simulink model "FlightSimulation"  (R2025b)
settings: Solver=ode3  StartTime=0.0  StopTime=100  FixedStep=params.time.dt  RelTol=1e-3
values from neighbouring files (symbols this model uses):
  launch_ECEF_m = lla2ecef(launchLLA)    [RunSim.m]    (also in RunSimulink.m)
  launchAlt = 180    [RunSim.m]    (also in RunSimulink.m = 10)
  launchLLA = [launchLat, launchLon, launchAlt]    [RunSim.m]    (also in RunSimulink.m)
  q = q / norm(q)    [CorrectQuaternionKinematics.m]    (also in solveLQR.m = 0.5*rho*vel^2)
  q_TB_0 = dcm2quat(R_TB_0)    [RunSimulink.m]
  w_ib_x = 0.00    (= 0)    [RunSim.m]    (also in RunSimulink.m = 1e-10)
  w_ib_y = 0.00    (= 0)    [RunSim.m]    (also in RunSimulink.m = 1e-10)
  w_ib_z = 0.00    (= 0)    [RunSim.m]    (also in RunSimulink.m = 1e-10)
undefined symbols (not defined in the file or in its folder): Earth, F, kfConsts, kfErrInds, kfInds, launchGeoidHeight, Light, MIL, nav_covs, nav_state, params, WGS84, WMM2025
libraries: simulink x6, aerolibatmos2 x5, aerolibgravity2 x3, aerolib6dof2 x1, aerolibwind2 x1, simulink_extras x1, matrix_library x1, aerolibtransform2 x1, lib_utils x1
(part 2 of 2)

== system FlightSimulation/Flight Computer/UKF/Update Step/GPS Update ==
  SensorBus : Inport
  navBus : Inport  Port=2
  Enable : EnablePort
  Bus Selector : BusSelector  OutputSignals=MAX10S.P_T
  MATLAB Function : MATLAB Function  TreatAsAtomicUnit=on
  navOut : Outport
  wires:
  MATLAB Function/1(navOut) -> navOut/1
  navBus/1 -> MATLAB Function/1(navIn)
  SensorBus/1 -> Bus Selector/1
  Bus Selector/1 -> MATLAB Function/2(u_k)  "<P_T>"

== system FlightSimulation/Flight Computer/UKF/Update Step/Gravity Update ==
  navBus : Inport
  SensorBus : Inport  Port=2
  Enable : EnablePort
  Bus Selector : BusSelector  OutputSignals=ICM20948.sf_B_corr
  MATLAB Function : MATLAB Function  TreatAsAtomicUnit=on
  navOut : Outport
  wires:
  navBus/1 -> MATLAB Function/1(navIn)
  SensorBus/1 -> Bus Selector/1
  Bus Selector/1 -> MATLAB Function/2(accelMeas)  "<sf_B_corr>"
  MATLAB Function/1(navOut) -> navOut/1

== system FlightSimulation/Flight Computer/UKF/Update Step/Mag Update ==
  SensorBus : Inport
  navBus : Inport  Port=2
  Enable : EnablePort
  Bus Selector : BusSelector  OutputSignals=MMC5983.B_corr
  MATLAB Function : MATLAB Function  TreatAsAtomicUnit=on
  navOut : Outport
  wires:
  MATLAB Function/1(navOut) -> navOut/1
  navBus/1 -> MATLAB Function/1(navIn)
  SensorBus/1 -> Bus Selector/1
  Bus Selector/1 -> MATLAB Function/2(u_mag)  "<B_corr>"

== matlab function FlightSimulation/Flight Computer/InertialSensors/MATLAB Function1 ==
  data: u input; y output
function y = fcn(u)

y = u;

== matlab function FlightSimulation/Flight Computer/Sensor Bus/ICM20948/MATLAB Function ==
  data: a_b input; sf_true output; R_BT input
function sf_true = accel2sf_(a_b, R_BT)

sf_true = accel2sf(a_b, R_BT);

== matlab function FlightSimulation/Flight Computer/Sensor Bus/ICM20948/MATLAB Function 1 ==
  data: sf_true input; sf_corr output; rn input
function sf_corr = corruptSensorReading(sf_true, rn)

ICM20948_PARAMS = getICM20948Params();


sf_corr = applySensorModel(sf_true, ICM20948_PARAMS.accel, rn);

== matlab function FlightSimulation/Flight Computer/Sensor Bus/MATLAB Function1 ==
  data: B_true input; B_corr output; rn input
function B_corr = corruptSensorReading(B_true, rn)

MMC5983_PARAMS = getMMC5983Params();

B_corr = applySensorModel(B_true, MMC5983_PARAMS, rn);

== matlab function FlightSimulation/Flight Computer/UKF/Update Step/GPS Update/MATLAB Function ==
  data: navIn input Bus: kfParamsBus; navOut output Bus: kfParamsBus; kfInds parameter; kfErrInds parameter; kfConsts parameter; u_k input; time parameter
function navOut = gpsUpdate(navIn, kfInds, kfErrInds, kfConsts, u_k, time)

    % Force column
    u_k = u_k(:);
    navOut = navIn;

    %% === Setup ===
    x_pred = navOut.x;
    P_min  = navOut.P;

    % Measurement model: position only
    z = u_k(1:3);                  % GPS position measurement
    h = x_pred(kfInds.pos);        % Predicted position
    y = z - h;                     % Innovation

    %% === Measurement Jacobian wrt error state ===
    H = zeros(3, kfErrInds.maxStateIndex);
    H(:, kfErrInds.pos) = eye(3);  % Only sensitive to position errors

    %% === Kalman Update ===
    R = kfConsts.R_gps;  % Should be 3x3 covariance of GPS measurement
    S = H * P_min * H' + R;
    K = P_min * H' / S;

    dx = K * y;  % Error state correction

    %% === Apply Correction to Nominal State ===
    x_update = x_pred;

    % Apply additive position correction
    x_update(kfInds.pos) = x_update(kfInds.pos) + dx(kfErrInds.pos);

    % Optional: could add velocity or clock bias terms here if needed

    % Apply corrected state
    navOut.x = x_update;

    % Joseph form update (for stability)
    I = eye(size(P_min));
    navOut.P = I - K * H;
    navOut.P = navOut.P * P_min * navOut.P' + K * R * K';
    navOut.P = 0.5 * (navOut.P + navOut.P');  % Enforce symmetry

end

== matlab function FlightSimulation/Flight Computer/Perfect TRIAD, GPS/MATLAB Function ==
  data: newState output; PrevState input; new_pos input; new_q input
function newState = fcn(PrevState, new_pos, new_q)



newState = PrevState;
newState(8:10) = new_pos;
%disp(PrevState(1:4))

    newState(1:4) = new_q';

== matlab function FlightSimulation/Flight Computer/UKF/Update Step/Mag Update/MATLAB Function ==
  data: navIn input Bus: kfParamsBus; navOut output Bus: kfParamsBus; kfInds parameter; kfErrInds parameter; kfConsts parameter; u_mag input
function navOut = magHeadingUpdate(navIn, kfInds, kfErrInds, kfConsts, u_mag)
    navOut = navIn;

    %% === Setup ===
    x_pred = navOut.x;
    P_min  = navOut.P;

    q  = x_pred(kfInds.quat);         % [w x y z]
    bm = x_pred(kfInds.magBias);      % Magnetometer bias

    %% === Measured field in body frame (bias corrected, normalized)
    m_b = u_mag(:) - bm;
    m_b = m_b / norm(m_b + 1e-8);  % normalize with epsilon to avoid NaNs

    %% === Rotate to NED and project to horizontal plane
    R_BN = quat2rotm(q');             % Body-to-NED
    m_n = R_BN * m_b;
    m_n(3) = 0;

    if norm(m_n) < 1e-3
        return;  % Insufficient horizontal component to resolve heading
    end

    m_n = m_n / norm(m_n);
    yaw_meas = atan2(-m_n(2), m_n(1));  % Heading in NED frame (E/N)

    %% === Predicted yaw from current quaternion
    qw = q(1); qx = q(2); qy = q(3); qz = q(4);
    yaw_pred = atan2(2*(qw*qz + qx*qy), 1 - 2*(qy^2 + qz^2));

    %% === Innovation ===
    y = wrapToPi(yaw_meas - yaw_pred);

    %% === Jacobian: ∂yaw/∂(δθ)
    dq = 1e-5;
    H_theta = zeros(1, 3);
    for i = 1:3
        dtheta = zeros(3,1);
        dtheta(i) = dq;
        dq_pert = smallAngleQuaternion(dtheta);
        q_pert = quatmultiply(dq_pert', q')';
        R_pert = quat2rotm(q_pert');
        m_n_pert = R_pert * m_b;
        m_n_pert(3) = 0;
        if norm(m_n_pert) < 1e-3
            return;
        end
        m_n_pert = m_n_pert / norm(m_n_pert);
        yaw_pert = atan2(-m_n_pert(2), m_n_pert(1));
        H_theta(i) = (yaw_pert - yaw_pred) / dq;
    end

    %% === Jacobian: ∂yaw/∂(bm)
    H_bm = zeros(1, 3);
    for i = 1:3
        db = zeros(3,1);
        db(i) = dq;
        m_b_pert = (u_mag(:) - bm - db);  % Subtract db for ∂h/∂bm = -∂h/∂m_b
        m_b_pert = m_b_pert / norm(m_b_pert + 1e-8);
        m_n_pert = R_BN * m_b_pert;
        m_n_pert(3) = 0;
        if norm(m_n_pert) < 1e-3
            return;
        end
        m_n_pert = m_n_pert / norm(m_n_pert);
        yaw_pert = atan2(-m_n_pert(2), m_n_pert(1));
        H_bm(i) = (yaw_pert - yaw_pred) / dq;
    end

    %% === Assemble Kalman update ===
    H = zeros(1, kfErrInds.maxStateIndex);
    H(1, kfErrInds.theta) = H_theta;
    H(1, kfErrInds.magBias) = H_bm;

    R = deg2rad(3)^2;  % 3 deg stddev → variance

    S = H * P_min * H' + R;
    K = P_min * H' / S;
    dx = K * y;

    %% === Apply correction to nominal state ===
    delta_q = smallAngleQuaternion(dx(kfErrInds.theta));
    q_update = quatmultiply(delta_q', q')';
    q_update = q_update / norm(q_update);

    x_update = x_pred;
    x_update(kfInds.quat)     = q_update;
    x_update(kfInds.magBias)  = x_update(kfInds.magBias) + dx(kfErrInds.magBias);

    navOut.x = x_update;

    %% === Covariance Update (Joseph Form) ===
    I = eye(size(P_min));
    navOut.P = (I - K * H) * P_min * (I - K * H)' + K * R * K';
    navOut.P = 0.5 * (navOut.P + navOut.P');  % Force symmetry
end

== matlab function FlightSimulation/Flight Computer/Sensor Bus/MATLAB Function2 ==
  data: h input; P_true output; const parameter; P_corr output; geoid_height input; rn input
function [P_true, P_corr] = corruptBarometer(h, const, geoid_height, rn)

rng(42);

LPS22_PARAMS = getLPS22HHParams();

P_true = height2baro(h, geoid_height);

bias = LPS22_PARAMS.bias;
noise = LPS22_PARAMS.noise;
sf   = LPS22_PARAMS.sf;
k2   = LPS22_PARAMS.k2;
k3   = LPS22_PARAMS.k3;

P_corr = height2baro(h + bias + (noise * rn), geoid_height);

== matlab function FlightSimulation/Flight Computer/UKF/Update Step/Baro Update/MATLAB Function ==
  data: navIn input Bus: kfParamsBus; navOut output Bus: kfParamsBus; kfInds parameter; kfConsts parameter; u_baro input; const parameter
function navOut = magHeadingUpdate(navIn, kfInds, kfConsts, u_baro, const)
    navOut = navIn;

    if any(isnan(navOut.x_pred))
        navOut.x = navOut.x_pred;
        navOut.P = navOut.P_min;
        return;
    end

    %% === Setup ===
    x_pred = navOut.x;
    P_min  = navOut.P;

    % Convert Pressure to Altitude
    h_baro = (const.T0 / const.L) * (1 - (u_baro / const.P0)^(const.R * const.L / const.g_e));

    z_pred = x_pred(kfInds.pos(3));
    h_pred = -h_baro;

    % Innovation
    y = h_baro - h_pred;

    %% Measurement Jacobian
    H = zeros(1, length(x_pred));
    H(kfInds.pos(3)) = -1;

    % Measurement Noise
    R_baro = (0.3)^2; % [m]

    % Kalman Gain and Update
    S = H * P_min * H' + R_baro;
    K = P_min * H' / S;

    x_update = x_pred + K * y;
    navOut.x = x_update;

    P_update = (eye(length(x_pred)) - K * H) * P_min;
    navOut.P = 0.5 * (P_update + P_update');
    

end

== matlab function FlightSimulation/Flight Computer/Sensor Bus/ICM20948/MATLAB Function 2 ==
  data: gyro_true input; gyro_corr output; rn input
function gyro_corr = corruptSensorReading(gyro_true, rn)

ICM20948_PARAMS = getICM20948Params();


gyro_corr = applySensorModel(gyro_true, ICM20948_PARAMS.gyro, rn);

== matlab function FlightSimulation/Flight Computer/Perfect TRIAD, GPS/MATLAB Function1 ==
  data: u input; y output
function y = fcn(u)

y = u;

== matlab function FlightSimulation/Flight Computer/Perfect TRIAD, GPS/MATLAB Function2 ==
  data: a_b input; R_TB output; m_b input; a_i input; m_i input
function R_TB = fcn(a_b, m_b, a_i, m_i)
R_TB = computeInitialQuaternionTRIAD(a_b, m_b, a_i, m_i);

== matlab function FlightSimulation/Flight Computer/Perfect TRIAD, GPS/g->sf ==
  data: u input; y output
function y = fcn(u)

y = u;
y(3) = -1.0 * y(3);

== matlab function FlightSimulation/Flight Computer/UKF/Initialize Nav/Initialize State/MATLAB Function2 ==
  data: a_b input; q_0 output; m_b input
function q_0 = computeInitialQuaternion_(a_b, m_b)

    q_0 = NaN(4,1);

    if((norm(a_b) > 1))
        q_0(1:4) = computeInitialQuaternion(a_b, m_b);
    end

== matlab function FlightSimulation/Flight Computer/UKF/Initialize Nav/Initialize State/MATLAB Function3 ==
  data: initFlagLoop input; q_0 input; x_0 output; navInds parameter; navParams parameter; initFlag output
function [x_0, initFlag]= initializeState_(initFlagLoop, q_0, navInds, navParams)
%#codegen

    x_0 = navParams.x;

    if(initFlagLoop == 1)
        initFlag = 1;
        return;
    end

    if any(isnan(q_0))
        initFlag = 0;
    
    else 
        x_0(navInds.quat) = q_0;
        initFlag = 1;
    end

== stateflow chart FlightSimulation/Flight Computer/Nav State Machine/Chart ==
  state PreLaunch
  state Launch
    entry:
    state=1
    guid=0
  state Burnout
    entry:
    state=2
    guid=0
  state Guidance
    entry:
    state=3
    guid=1
  state Apogee
    entry:
    state=4
    guid=0
  (default) -> PreLaunch : {state=0}
  PreLaunch -> Launch : [A_b_x > 3]
  Launch -> Burnout : [A_b_x < 1]
  Burnout -> Guidance : [after(1, sec)]
  Guidance -> Apogee : [v_vert < 1]
  data: A_b_x input; alt input; v_vert input; guid output; state output

== matlab function FlightSimulation/Flight Computer/UKF/Update Step/Gravity Update/MATLAB Function ==
  data: navIn input Bus: kfParamsBus; navOut output Bus: kfParamsBus; kfInds parameter; kfErrInds parameter; kfConsts parameter; accelMeas input
function navOut = gravityUpdate(navIn, kfInds, kfErrInds, kfConsts, accelMeas)
    g = 9.80665;  % Gravity magnitude
    navOut = navIn;

    if any(isnan(navOut.x_pred))
        navOut.x = navOut.x_pred;
        navOut.P = navOut.P_min;
        return;
    end

    %% === Setup ===
    x_pred = navOut.x_pred;
    P_min  = navOut.P_min;

    q  = x_pred(kfInds.quat);        % Quaternion: body-to-NED
    ba = x_pred(kfInds.accelBias);   % Accel bias

    G_NED = [0; 0; g];               
    R_NB = quat2rotm(q');            % Rotation body-to-NED

    %% === Measurement Prediction ===
    accel_pred = R_NB' * G_NED + ba;
    accel_meas = accelMeas(:);
    
    % Optional: Skip update if dynamic
    if abs(norm(accel_meas) - g) > 1.0
        return;
    end

    y = accel_meas - accel_pred;

    %% === Jacobian ===
    H = zeros(3, kfErrInds.maxStateIndex);
    H(:, kfErrInds.theta)     = -R_NB * skew(G_NED);
    H(:, kfErrInds.accelBias) = eye(3);

    R = kfConsts.R_grav;

    %% === Kalman Update ===
    S = H * P_min * H' + R;
    K = P_min * H' / S;
    dx = K * y;

    %% === Apply Correction ===
    delta_theta = dx(kfErrInds.theta);
    angle = norm(delta_theta);
    if angle > deg2rad(10)
        delta_theta = delta_theta * (deg2rad(10) / angle);
    end

    delta_q = smallAngleQuaternion(delta_theta);
    q_update = quatmultiply(delta_q', q')';  % delta_q ⊗ q

    x_update = x_pred;
    x_update(kfInds.quat)       = q_update / norm(q_update);  
    x_update(kfInds.accelBias)  = x_update(kfInds.accelBias) + dx(kfErrInds.accelBias);

    %% === Covariance Update ===
    I = eye(size(P_min));
    P_update = (I - K * H) * P_min * (I - K * H)' + K * R * K'; 

    navOut.x = x_update;
    navOut.P = 0.5 * (P_update + P_update');  % Ensure symmetry
end

== matlab function FlightSimulation/Flight Computer/UKF/Update Step/MATLAB Function ==
  data: navOut output Bus: navBus; navIn input Bus: navBus
function navOut = passiveUpdate(navIn)

navOut = navIn;

navOut.x = navOut.x_min;
navOut.P = navOut.P_min;

navOut.P = (navOut.P + navOut.P') * 0.5;

== matlab function FlightSimulation/Flight Computer/Perfect TRIAD, GPS/Switch statement bruh why do i gotta make a matlab func for this ==
  data: a_b input; p_b output; a_i input; v_b input; v_i input; State input; p_i output
function [p_b, p_i] = fcn(a_b, a_i, v_b, v_i, State)
if State > 0 && State < 4
    p_b = v_b;
    p_i = v_i;
else
    p_b = a_b;
    p_i = a_i;
end

== matlab function FlightSimulation/Flight Computer/Perfect TRIAD, GPS/MATLAB Function3 ==
  data: u input; y output
function y = fcn(u)

y = [norm(u); 0; 0];

== matlab function FlightSimulation/Flight Computer/ESKF/GPS update ==
  settings: updateMethod=DISCRETE
  data: curr_state input; new_state output size=[20, 1]; curr_P input; State input; gps_pos_meas input; gps_vel_meas input; new_P output; time input
function [new_state, new_P] = fcn(curr_state, curr_P, State, gps_pos_meas, gps_vel_meas, time)
new_state = curr_state;
new_P = curr_P;


if (time > 0.1 && State ~= 1)
    GPS_PARAMS = getMAX10SParams();
    z = [gps_pos_meas; gps_vel_meas];
    h = [curr_state(8:10); curr_state(5:7)];
    H = [zeros(3, 6), eye(3, 3), zeros(3, 10);
        zeros(3, 3), eye(3, 3), zeros(3, 13)];
    R = diag([GPS_PARAMS.pos.noise; GPS_PARAMS.vel.noise]);
    
    [new_state, new_P] = residualErrInject(curr_state, curr_P, z, H, h, R);
end

end

== matlab function FlightSimulation/Flight Computer/ESKF/Accel+Mag update ==
  settings: updateMethod=DISCRETE
  data: curr_state input; new_state output; curr_P input; State input; accel_meas input; accel_inertial input; new_P output; mag_meas input; mag_inertial input; time input
function [new_state, new_P] = fcn(curr_state, curr_P, State, accel_meas, accel_inertial, mag_meas, mag_inertial, time)
new_state = curr_state;
new_P = curr_P;

MAG_PARAMS = getMMC5983Params();
ACCEL_PARAMS = getICM20948Params().accel;

q = curr_state(1:4)';

if (State == 0 && time > 0.1)

    rec_accel_body = quat2rotm(q)' * accel_inertial;
    rec_mag_body = quat2rotm(q)' * mag_inertial;
    
    
    z = [accel_meas; mag_meas];
    h = [rec_accel_body; rec_mag_body];
    H = [skewSymmetric(rec_accel_body), zeros(3, 9), eye(3, 3), zeros(3, 4);
        skewSymmetric(rec_mag_body), zeros(3, 12), eye(3, 3), zeros(3, 1)];
    R = diag([ACCEL_PARAMS.noise; MAG_PARAMS.noise]);
    
    [new_state, new_P] = residualErrInject(curr_state, curr_P, z, H, h, R);
else

end

== matlab function FlightSimulation/Flight Computer/ESKF/MATLAB Function2 ==
  data: a_b input; R_TB output; m_b input; a_i input; m_i input
function R_TB = fcn(a_b, m_b, a_i, m_i)
R_TB = computeInitialQuaternionTRIAD(a_b, m_b, a_i, m_i);

== matlab function FlightSimulation/Flight Computer/ESKF/MATLAB Function3 ==
  data: u input; y output
function y = fcn(u)

y = [norm(u); 0; 0];

== matlab function FlightSimulation/Flight Computer/UKF/Initialize Nav/Initialize State/MATLAB Function1 ==
  data: a_b input; eul_0 output; m_b input
function eul_0 = computeInitialOrientation_(a_b, m_b)

    % q_0 = NaN(4,1);
    eul_0 = NaN(3,1);

    if((norm(a_b) > 0.5))
        eul_0(1:3) = computeInitialOrientation(a_b, m_b);
    end

== matlab function FlightSimulation/Flight Computer/ESKF/Switch statement bruh why do i gotta make a matlab func for this ==
  data: a_b input; p_b output; a_i input; v_b input; v_i input; State input; p_i output
function [p_b, p_i] = fcn(a_b, a_i, v_b, v_i, State)
if State > 0 && State < 4
    p_b = v_b;
    p_i = v_i;
else
    p_b = a_b;
    p_i = a_i;
end

== matlab function FlightSimulation/Flight Computer/ESKF/g->sf ==
  data: u input; y output
function y = fcn(u)

y = u;
y(3) = -1.0 * y(3);

== matlab function FlightSimulation/Flight Computer/ESKF/Propagate non-linear dynamics aka fast gyro+accel prop ==
  data: gyro input; newState output; PrevState input; dt input; accel input; g_i input
function newState = fcn(gyro, PrevState, dt, accel, g_i)


prev_quat = quaternion(PrevState(1:4)');
prev_pos = PrevState(8:10);
prev_vel = PrevState(5:7);


newState = PrevState;

new_quat = propGyro(gyro, prev_quat, dt);
[new_pos, new_vel] = propAccel(accel, prev_vel, prev_pos, new_quat, g_i, dt);

newState(1:4) = new_quat;
newState(5:7) = new_vel;
newState(8:10) = new_pos;

== matlab function FlightSimulation/Flight Computer/ESKF/Predict Covs aka ekf predict ==
  settings: updateMethod=DISCRETE
  data: gyro input; curr_P output; accel input; prev_P input; curr_state input; dt input
function curr_P = fcn(gyro, accel, prev_P, curr_state, dt)

IMU_PARAMS = getICM20948Params();
MAG_PARAMS = getMMC5983Params();
BARO_PARAMS = getLPS22HHParams();


curr_quat = quaternion(curr_state(1:4)');

curr_P = predictCovariances(gyro, accel, prev_P, curr_quat, dt, IMU_PARAMS.gyro, IMU_PARAMS.accel, MAG_PARAMS, BARO_PARAMS);

== matlab function FlightSimulation/Flight Computer/ESKF/Baro update ==
  settings: updateMethod=DISCRETE
  data: curr_state input; new_state output; curr_P input size=[19, 19]; State input; baro_meas input; geoid_height input; launchAlt input; new_P output size=[19, 19]; time input; baro_height output
function [new_state, new_P, baro_height] = fcn(curr_state, curr_P, State, baro_meas, geoid_height, launchAlt, time)
new_state = curr_state;
new_P = curr_P;
baro_height = 0;

if (time > 0.1)
    BARO_PARAMS = getLPS22HHParams();
    
    baro_height = -1.0 * ((baro2height(baro_meas, geoid_height) - launchAlt) + curr_state(20));
    %disp("Baro height")
    %disp(time)
    %disp(baro_height)
    %disp("End")
    
    z = baro_height;
    h = [curr_state(10)];
    H = [zeros(1, 8), 1, zeros(1, 9), 1.0]; % TODO eventually add baro bias
    R = BARO_PARAMS.noise;
    [new_state, new_P] = residualErrInject(curr_state, curr_P, z, H, h, R);
end

end

== matlab function FlightSimulation/Flight Computer/ESKF/Unbias sensors ==
  data: w_ib_b_biased input; w_ib_b output; sf_b_biased input; B_biased input; LLA_biased input; V_T_biased input; P_biased input; prev_state input; sf_b output; B output; LLA output; V_T output; P output
function [w_ib_b, sf_b, B, LLA, V_T, P] = fcn(w_ib_b_biased, sf_b_biased, B_biased, LLA_biased, V_T_biased, P_biased, prev_state)

w_ib_b = w_ib_b_biased - prev_state(11:13);
sf_b = sf_b_biased - prev_state(14:16);
B = B_biased - prev_state(17:19);
LLA = LLA_biased;
V_T = V_T_biased;
%P = P_biased - prev_state(20);
P = P_biased;

== matlab function FlightSimulation/Flight Computer/UKF/Prediction Step/MATLAB Function ==
  data: navOut output Bus: navBus; navIn input Bus: navBus; sf_b input; w_ib_b input; time parameter; navInds parameter; navParams parameter
function navOut = UKFPredict(navIn, sf_b, w_ib_b, time, navInds, navParams)

dt = time.navDt;

% === Format Input ===
u = [w_ib_b(:); sf_b(:)];

navOut = navIn;

%% === GENERATE SIGMA POINTS ===
[X_sigma, P_sigma] = unscentedSigmaPoints(navIn.x, navIn.P, navParams.lambda);

X_sigma_pred = processModel(X_sigma, u, dt, navInds);

[x_min, P_min] = unscentedMeanCov(X_sigma_pred, navIn.W_m, navIn.W_c, navParams.Q);

navOut.x_min  = x_min;
navOut.P_min  = P_min;

% persistent ukf
% 
% if(isempty(ukf))
%     dynamicsFunc = @(x, dt, u) ukfDynamics(x, dt, u, navInds);
%     ukf = StavUKF(dynamicsFunc, navIn.Q);
% end
% 

% 
% % === Prepare State Struct ===
% stateStruct.mean = navIn.x;
% stateStruct.cov  = navIn.P;
% 
% % === UKF Prediction Step ===
% [prior, sigma] = ukf.predict(stateStruct, dt, u);
% 
% sigPts = sigma.sigmaPts;

% === Fill Output Bus ===
% navOut.x_min = prior.mean;
% navOut.P_min  = prior.cov;

== stateflow chart FlightSimulation/Flight Computer/State Machine/Chart ==
  state PreLaunch
  state Launch
    entry:
    state=1
    guid=0
  state Burnout
    entry:
    state=2
    guid=0
  state Guidance
    entry:
    state=3
    guid=1
  state Apogee
    entry:
    state=4
    guid=0
  (default) -> PreLaunch : {state=0}
  PreLaunch -> Launch : [A_b_x > 3]
  Launch -> Burnout : [A_b_x < 1]
  Burnout -> Guidance : [after(1, sec)]
  Guidance -> Apogee : [v_vert < 1]
  data: A_b_x input; alt input; v_vert input; guid output; state output; v_b input

== matlab function FlightSimulation/Flight Computer/UKF/Initialize Nav/Initialize State/MATLAB Function4 ==
  data: initFlagLoop input; eul_0 input; x_0 output; navInds parameter; navParams parameter; initFlag output
function [x_0, initFlag]= initializeState_(initFlagLoop, eul_0, navInds, navParams)
%#codegen

    x_0 = navParams.x;

    if(initFlagLoop == 1)
        x_0(navInds.eul) = eul_0;
        initFlag = 1;
        return;
    end

    if any(isnan(eul_0))
        initFlag = 0;
    else 
        x_0(navInds.eul) = eul_0;
        initFlag = 1;
    end

== matlab function FlightSimulation/Flight Computer/Const/MATLAB Function ==
  data: u input; y output
function y = fcn(u)

y = zeros(19, 1);

== matlab function FlightSimulation/Flight Computer/Const/MATLAB Function1 ==
  data: u input; y output
function y = fcn(u)

y = eye(22);

== matlab function FlightSimulation/Flight Computer/InertialSensors/MATLAB Function ==
  data: gyro input; newState output; PrevState input; dt input; accel input; g_i input
function newState = fcn(gyro, PrevState, dt, accel, g_i)


prev_quat = quaternion(PrevState(1:4)');
prev_pos = PrevState(8:10);
prev_vel = PrevState(5:7);


newState = PrevState;

new_quat = propGyro(gyro, prev_quat, dt);
[new_pos, new_vel] = propAccel(accel, prev_vel, prev_pos, new_quat, g_i, dt);

newState(1:4) = new_quat;
newState(5:7) = new_vel;
newState(8:10) = new_pos;
